simulink model "valmotor"  (Simulink 4.00)
settings: Solver=ode45  StartTime=0.0  StopTime=0.9  MaxStep=1/80000  RelTol=1e-3
settings Model: LastModifiedBy=Gui

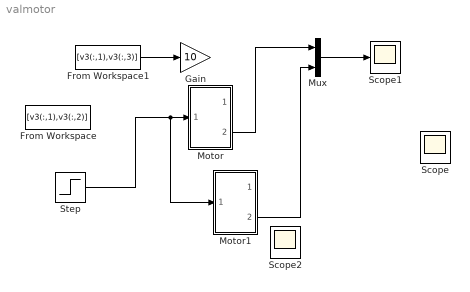
== system valmotor ==
  From Workspace : FromWorkspace  VariableName=[v3(:,1),v3(:,2)]  SampleTime=0  OutputAfterFinalValue=Extrapolation
  From Workspace1 : FromWorkspace  VariableName=[v3(:,1),v3(:,3)]  SampleTime=0  OutputAfterFinalValue=Extrapolation
  Gain : Gain  Gain=10  Multiplication=Element-wise(K.*u)  SaturateOnIntegerOverflow=on
  Motor : Subsystem
      settings: RTWFcnNameOpts=Auto  RTWFileNameOpts=Auto
  Motor1 : Subsystem
      settings: RTWFcnNameOpts=Auto  RTWFileNameOpts=Auto
  Mux : Mux  Inputs=3
  Scope : Scope
      settings: TimeRange=auto  YMin=-5  YMax=5  SaveToWorkspace=off  SaveName=ScopeData  MaxDataPoints=5000
  Scope1 : Scope
      settings: TimeRange=0.045  YMin=251.775  YMax=252.175  SaveName=corr  MaxDataPoints=5000
  Scope2 : Scope
      settings: TimeRange=auto  YMin=-5  YMax=5  SaveToWorkspace=off  SaveName=ScopeData2  MaxDataPoints=5000
  Step : Step  Time=0  Before=0  After=12  SampleTime=0
  wires:
  Mux/1 -> Scope1/1
  From Workspace1/1 -> Gain/1
  Motor/2(Out2) -> Mux/1
  Motor1/2(Out2) -> Mux/3
  Step/1 -> Motor/1(In1), Motor1/1(In1)

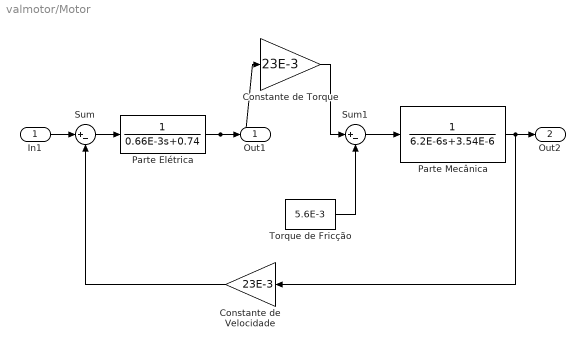
== system valmotor/Motor ==
  In1 : Inport  Port=1  LatchInput=off
  Constante de Torque : Gain  Gain=23E-3  Multiplication=Element-wise(K.*u)  SaturateOnIntegerOverflow=on
  Constante de Velocidade : Gain  Orientation=left  Gain=23E-3  Multiplication=Element-wise(K.*u)  SaturateOnIntegerOverflow=on
  Parte Elétrica : TransferFcn  Numerator=[1]  Denominator=[0.66E-3 0.74]  AbsoluteTolerance=auto  Realization=auto
  Parte Mecânica : TransferFcn  Numerator=[1]  Denominator=[6.2E-6 3.54E-6]  AbsoluteTolerance=auto  Realization=auto
  Sum : Sum  Inputs=|+-  SaturateOnIntegerOverflow=on
  Sum1 : Sum  Inputs=|+-  SaturateOnIntegerOverflow=on
  Torque de Fricção : Constant  Value=5.6E-3
  Out1 : Outport  Port=1
  Out2 : Outport  Port=2
  wires:
  Sum/1 -> Parte Elétrica/1
  Parte Elétrica/1 -> Constante de Torque/1, Out1/1
  Parte Mecânica/1 -> Constante de Velocidade/1, Out2/1
  Constante de Velocidade/1 -> Sum/2
  Constante de Torque/1 -> Sum1/1
  Sum1/1 -> Parte Mecânica/1
  Torque de Fricção/1 -> Sum1/2
  In1/1 -> Sum/1

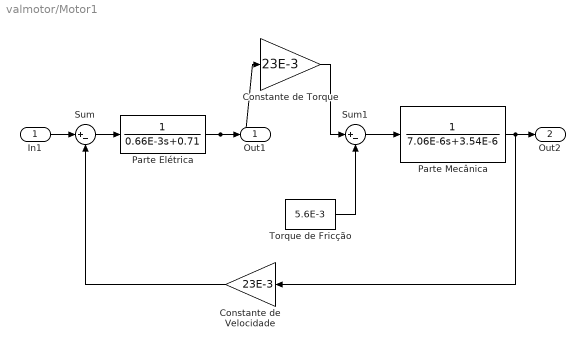
== system valmotor/Motor1 ==
  In1 : Inport  Port=1  LatchInput=off
  Constante de Torque : Gain  Gain=23E-3  Multiplication=Element-wise(K.*u)  SaturateOnIntegerOverflow=on
  Constante de Velocidade : Gain  Orientation=left  Gain=23E-3  Multiplication=Element-wise(K.*u)  SaturateOnIntegerOverflow=on
  Parte Elétrica : TransferFcn  Numerator=[1]  Denominator=[0.66E-3 0.71]  AbsoluteTolerance=auto  Realization=auto
  Parte Mecânica : TransferFcn  Numerator=[1]  Denominator=[7.06E-6 3.54E-6]  AbsoluteTolerance=auto  Realization=auto
  Sum : Sum  Inputs=|+-  SaturateOnIntegerOverflow=on
  Sum1 : Sum  Inputs=|+-  SaturateOnIntegerOverflow=on
  Torque de Fricção : Constant  Value=5.6E-3
  Out1 : Outport  Port=1
  Out2 : Outport  Port=2
  wires:
  Sum/1 -> Parte Elétrica/1
  Parte Elétrica/1 -> Constante de Torque/1, Out1/1
  Parte Mecânica/1 -> Constante de Velocidade/1, Out2/1
  Constante de Velocidade/1 -> Sum/2
  Constante de Torque/1 -> Sum1/1
  Sum1/1 -> Parte Mecânica/1
  Torque de Fricção/1 -> Sum1/2
  In1/1 -> Sum/1
